simulink model "Ford_T3T6_ArchCnctnDigrm"  (R2016b)
settings: Solver=FixedStepDiscrete  StartTime=0.0  StopTime=10.0  RelTol=1e-3  EnableMultiTasking=on
libraries: canmsglib x15
(part 1 of 15)
Description:
  | T1xx system diagram for build 3
settings Model: SimulationMode=accelerator  Creator=xzs3wb  LastModifiedBy=nz3503
settings SolverCC: AutoInsertRateTranBlk=on
settings DataIOCC: LimitDataPoints=on  SaveFormat=Array  SignalLoggingSaveFormat=ModelDataLogs  SaveOutput=off  SaveTime=off
settings OptimizationCC: DefaultParameterBehavior=Inlined  InlineInvariantSignals=on  StateBitsets=on  DataBitsets=on  ZeroExternalMemoryAtStartup=off  ZeroInternalMemoryAtStartup=off  NoFixptDivByZeroProtection=on  LifeSpan=1
settings DebuggingCC: SaveWithParameterizedLinksMsg=none  UnderspecifiedInitializationDetection=Classic  MergeDetectMultiDrivingBlocksExec=none  SignalResolutionControl=TryResolveAllWithWarning  MultiTaskDSMMsg=warning  MultiTaskCondExecSysMsg=none  ParameterTunabilityLossMsg=error  StrictBusMsg=None  SFUnexpectedBacktrackingDiag=warning  SFNoUnconditionalDefaultTransitionDiag=warning  SFExecutionAtInitializationDiag=none
settings HardwareCC: ProdBitPerPointer=32  ProdBitPerSizeT=32  ProdBitPerPtrDiffT=32  ProdLargestAtomicFloat=None  ProdIntDivRoundTo=Floor  ProdWordSize=32  ProdHWDeviceType=Generic->Custom  TargetBitPerPointer=64  TargetBitPerSizeT=64  TargetBitPerPtrDiffT=64  TargetLongLongMode=on  TargetIntDivRoundTo=Zero  TargetEndianess=LittleEndian  TargetWordSize=64  TargetHWDeviceType=MATLAB Host  ProdEqTarget=off
settings ModelReferenceCC: PropagateSignalLabelsOutOfModel=off
settings RTWCC: SystemTargetFile=ert.tlc  TLCOptions=-p0  GenCodeOnly=on  TemplateMakefile=ert_default_tmf  Description=Embedded Coder  GenerateReport=on  RTWVerbose=off  IncludeHyperlinkInReport=on  LaunchReport=on  GenerateTraceInfo=on  GenerateTraceReport=on  GenerateTraceReportSl=on  GenerateTraceReportSf=on  GenerateTraceReportEml=on
settings CodeAppCC: ForceParamTrailComments=on  IgnoreCustomStorageClasses=off  OperatorAnnotations=on  SimulinkDataObjDesc=on  SFDataObjDesc=on  MATLABFcnDesc=on  CustomSymbolStrGlobalVar=rt$N$M  CustomSymbolStrType=$N$M  CustomSymbolStrFcn=$N$M$F  CustomSymbolStrMacro=$N$M  InsertBlockDesc=on  MATLABSourceComments=on
settings ERTTargetCC: CodeReplacementLibrary=ISO_C  GenerateSampleERTMain=on  IncludeMdlTerminateFcn=off  SuppressErrorStatus=on  SupportAbsoluteTime=off  SupportNonFinite=off  SupportComplex=off  PurelyIntegerCode=on  InlinedParameterPlacement=NonHierarchical  RootIOFormat=Structure reference  ERTCustomFileTemplate=example_file_process.tlc
settings ConfigComp: CovMetricSettings=dw  CovHtmlReporting=on  CovSaveCumulativeToWorkspaceVar=on  CovSaveSingleToWorkspaceVar=on  CovExternalEMLEnable=off

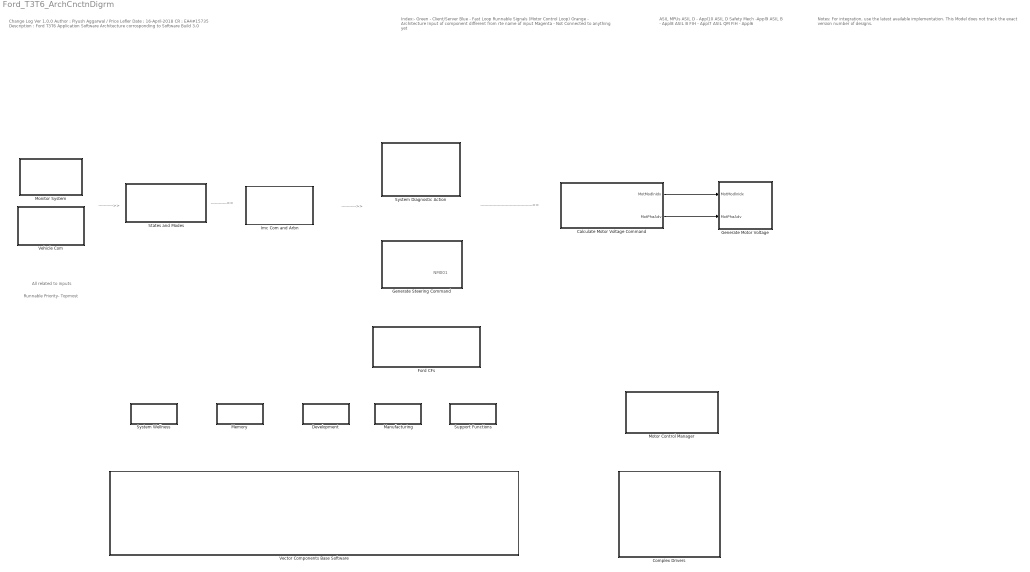
== system Ford_T3T6_ArchCnctnDigrm ==
  note: --------------------------------------->>
  note: Runnable Priority- Topmost
  note: All related to inputs
  note: ------------>>
  note: ----------->>
  note: ----------->>
  note: Change Log
      |
      | Ver 1.0.0
      | Author : Piyush Aggarwal / Price Lefler
      | Date : 16-April-2018
      | CR : EA4#15735
      | Description : Ford T3T6 Application Software Architecture corrosponding to Software Build 3.0
  note: Index:-
      |
      | Green - Client/Server
      | Blue - Fast Loop Runnable Signals (Motor Control Loop)
      | Orange - Architecture Input of component different from rte name of input
      | Magenta - Not Connected to anything yet
  note: ASIL MPUs
      |
      | ASIL D - Appl10
      | ASIL D Safety Mech -Appl9
      | ASIL B - Appl8
      | ASIL B FIH - Appl7
      | ASIL QM FIH - Appl6
  note: NM001
  note: Notes:
      | For integration, use the latest available implementation. This Model does not track the exact version number of designs.
  Calculate Motor Voltage Command : Subsystem
  Complex Drivers : Subsystem
  Development : Subsystem
  Ford CFs : Subsystem
  Generate Motor Voltage : Subsystem
  Generate Steering Command : Subsystem
  Imc Com and Arbn : Subsystem
  Manufacturing : Subsystem
  Memory : Subsystem
  Monitor System : Subsystem
  Motor Control Manager : Subsystem
  States and Modes : Subsystem
  Support Functions : Subsystem
  System Diagnostic Action : Subsystem
  System Wellness : Subsystem
  Vector Components Base Software : Subsystem
  Vehicle Com : Subsystem
  wires:
  Calculate Motor Voltage Command/1(MotModlnIdx) -> Generate Motor Voltage/1(MotModlnIdx)
  Calculate Motor Voltage Command/2(MotPhaAdv) -> Generate Motor Voltage/2(MotPhaAdv)

== system Ford_T3T6_ArchCnctnDigrm/Calculate Motor Voltage Command ==
  note: Diag Service?
  note: ASIL D
  note: ASIL D
  Motor Control : Subsystem
  SF019B_PwrLimr : Subsystem  Tag=4.0.0  Description="The purpose of the Power Limit function is to limit the system output power in a manner to enforce a desired limit on the system supply current draw.  The Power Limit function limits system output power as a function of available voltage at the inverter (DC Link Voltage) and Motor Velocity.  Additionally, a function is included to prevent excessive motor currents from being requested when the system is very hot (i.e., in Extended Operating Conditions for temperature). In additional to calculation of the Power Limit, the Power Limit Function also calculates a level of degradation from Standard Operating Conditions full performance and sets flags appropriately for a DTC (Log Only). *** PosSrvoEnable_Cnt_lgc is in documentation, but not in code. ***"
      settings: AttributesFormatString=Version: %<Tag>
  SF032A_MotTqCmdSca1 : Subsystem  Tag=1.2.3  Description=The Torque Command Scale function multiplies the MRF Motor Torque Commandinput signal by a calibration which is set during a manufacturing end of line calibration process. The calibration is provided to reduce overall system outputtorque variation. This scaled version of the motor torque command is used by SF99B - Motor control
      settings: AttributesFormatString=Version: %<Tag>
  SF050A_MotTqTranlDampg : Subsystem  Tag=1.3.0  Description=Transitional damping is computed, triggered by LoaState or DiagStatus
      settings: AttributesFormatString=Version: %<Tag>
  MotModlnIdx : Outport
  MotPhaAdv : Outport  Port=2
  tag scope: GetMotTqCmdSca=global, MotTqCmdCrfDampd=global, MotTqCmdMrfScad=global, MotTqCmdPwrLimd=global, MotTqTranlDampgCmpl=global, PwrLimrRednFac=global, SetMotTqCmdSca=global
  wires:
  Motor Control/1(MotModlnIdx) -> MotModlnIdx/1
  Motor Control/2(MotPhaAdv) -> MotPhaAdv/1
  [AltFltActv] -> SF019B_PwrLimr/1(AltFltActv)
  [BrdgVltg] -> SF019B_PwrLimr/2(BrdgVltg)
  [DualEcuFltMtgtnSca] -> SF019B_PwrLimr/3(DualEcuFltMtgtnSca)
  [MotAndThermProtnLoaMod] -> SF019B_PwrLimr/4(MotAndThermProtnLoaMod)
  [MotBackEmfConEstimd] -> SF019B_PwrLimr/5(MotBackEmfConEstimd)
  SF050A_MotTqTranlDampg/2(MotTqCmdMrfDampd) -> SF019B_PwrLimr/6(MotTqCmdMrf)
  [MotVelMrf] -> SF019B_PwrLimr/7(MotVelMrf)
  [GetRefTmr100MicroSec32bit] -> SF019B_PwrLimr/8(GetRefTmr100MicroSec32bit)
  [GetTiSpan100MicroSec32bit] -> SF019B_PwrLimr/9(GetTiSpan100MicroSec32bit)
  [SetNtcSts10] -> SF019B_PwrLimr/10(SetNtcSts)
  SF019B_PwrLimr/2(PwrLimrRednFac) -> [PwrLimrRednFac]
  SF019B_PwrLimr/1(MotTqCmdPwrLimd) -> [MotTqCmdPwrLimd], SF032A_MotTqCmdSca1/1(MotTqCmdMrf)
  [NvMProxy_GetErrorStatus] -> SF032A_MotTqCmdSca1/2(MotTqScaFac_GetErrorStatus)
  [NvMProxy_SetRamBlockStatus] -> SF032A_MotTqCmdSca1/3(MotTqScaFac_SetRamBlockStatus)
  SF032A_MotTqCmdSca1/1(MotTqCmdMrfScad) -> Motor Control/1(MotTqCmdMrfFinal), [MotTqCmdMrfScad]
  SF032A_MotTqCmdSca1/2(GetMotTqCmdSca) -> [GetMotTqCmdSca]
  SF032A_MotTqCmdSca1/3(SetMotTqCmdSca) -> [SetMotTqCmdSca]
  [AssiMechPolarity] -> SF050A_MotTqTranlDampg/1(AssiMechPolarity)
  [DiagcStsCtrldShtDwnFltPrsnt] -> SF050A_MotTqTranlDampg/2(DiagcStsCtrldShtDwnFltPrsnt)
  [HwAg] -> SF050A_MotTqTranlDampg/3(HwAg)
  [LoaSt] -> SF050A_MotTqTranlDampg/4(LoaSt)
  [MotTqCmdSwp] -> SF050A_MotTqTranlDampg/5(MotTqCmdCrf)
  [MotVelCrf] -> SF050A_MotTqTranlDampg/6(MotVelCrf)
  [SysSt] -> SF050A_MotTqTranlDampg/7(SysSt)
  [VehSpd] -> SF050A_MotTqTranlDampg/8(VehSpd)
  [GetRefTmr100MicroSec32bit] -> SF050A_MotTqTranlDampg/9(GetRefTmr100MicroSec32bit)
  [GetTiSpan100MicroSec32bit] -> SF050A_MotTqTranlDampg/10(GetTiSpan100MicroSec32bit)
  SF050A_MotTqTranlDampg/1(MotTqCmdCrfDampd) -> [MotTqCmdCrfDampd]
  SF050A_MotTqTranlDampg/3(MotTqTranlDampgCmpl) -> [MotTqTranlDampgCmpl]

== system Ford_T3T6_ArchCnctnDigrm/Complex Drivers ==
  note: ASIL D Safety Mech.
  note: ASIL D Safety Mech.
  note: ASIL D
  note: ASIL D Safety Mech.
  note: ASIL D
  AR102B_NxtrTi : Subsystem  Tag=1.0.0  Description=Nexteer Time Library
      settings: AttributesFormatString=Version: %<Tag>
  CM101B_ExcpnHndlg : Subsystem  Tag=1.2.0  Description=Handles exceptions, FE server functions and sets pre OS start up faults
      settings: AttributesFormatString=Version: %<Tag>
  CM102B_FlsMem : Subsystem  Tag=1.1.0  Description=Code Flash memory diagnostics
      settings: AttributesFormatString=Version: %<Tag>
  CM103B_RamMem : Subsystem  Tag=1.1.0  Description=Diagnostics related to RAM memory - Local, periperal and I-Cache
      settings: AttributesFormatString=Version: %<Tag>
  CM104B_EcmOutpAndDiagc : Subsystem  Tag=1.2.0  Description=Manual control over error out pin (ERROROUTZ) and startup verification test of ECM Master/Checker functionality
      settings: AttributesFormatString=Version: %<Tag>
  CM106B_McuCoreCfgAndDiagc : Subsystem  Tag=1.1.0  Description=This function describes some of the basic MCU diagnostics of the RH850/P1MC microcontroller Field BIST (built-in self-test)
      settings: AttributesFormatString=Version: %<Tag>
  CM109B_ClkCfgAndMon : Subsystem  Tag=1.1.0  Description=Nexteer Clock Monitor Config And Use
      settings: AttributesFormatString=Version: %<Tag>
  CM800A_SyncCrc : Subsystem  Tag=1.2.0  Description=CM800A provides an API for software components to run synchronous CRC calculations with the hardware CRC units on the EA4 micro controller
      settings: AttributesFormatString=Version: %<Tag>
  ES104B_XcpIf : Subsystem  Tag=0.0.0  Description=[ ]
      settings: AttributesFormatString=Version: %<Tag>
  Ford001A_ChkPt : Subsystem  Tag=0.0.0  Description=Check Point Supports alive monitoring and program flow monitoring
      settings: AttributesFormatString=Version: %<Tag>
  Platform Config : Subsystem
  tag scope: Calc16BitCrc_u08=global, Calc16BitCrc_u16=global, Calc32BitCrc_u08=global, Calc32BitCrc_u16=global, Calc32BitCrc_u32=global, Calc8BitCrc0X2F=global, Calc8BitCrc=global, ChkForStrtUpTest=global, CodFlsCrcChkCmpl=global, CtrlErrOut=global, FeNmiBusBrdgErr=global, FeNmiBusSngBitEccErr=global, FeNmiClkMonr0RtErr=global, FeNmiClkMonr1RtErr=global, FeNmiClkMonr2RtErr=global, FeNmiClkMonr3RtErr=global, FeNmiClkMonr5RtErr=global, FeNmiCodFlsEccAdrOvfErr=global, FeNmiCodFlsIllglAcsBySysBus=global, FeNmiDmaIllglAcsErr=global, FeNmiDmaLockStepErrOrGblRamWrBufErr=global, FeNmiDmaTrfErr=global, FeNmiDtsRamDblBitEccErr=global, FeNmiEcmMstChkrErr=global, FeNmiFlsSeqErr=global, FeNmiGblRamIllglAcsByProcr=global, FeNmiGblRamIllglAcsBySysBus=global, FeNmiGlbRamEccAdrOvfErr=global, FeNmiGtmRamDblBitEccErr=global, FeNmiLclRamEccAdrOvfErr=global, FeNmiModErrDbgActv=global, FeNmiModErrProgmModActv=global, FeNmiModErrTestModActv=global, FeNmiModErrUsrModInactv=global, FeNmiPegErr=global, FeNmiProcrLockStepErr=global, FeNmiPrphlRamEccAdrOvfErr=global, FeNmiResdAreaIllglAcsByHiSpdBus=global, FeNmiWdgErr=global, GetMcuDiagcIdnData=global, GetMcuDiagcSpplData=global, GetRefTmr100MicroSec32bit=global, GetRefTmr1MicroSec32bit=global, GetTiSpan100MicroSec32bit=global, GetTiSpan1MicroSec32bit=global, GlbRamEccSngBitCntrOutp=global, LclRamEccSngBitCntrOutp=global, ProcMpuExcpnErr=global, ProcNonCritOsErr=global, ProcPrmntOsErr=global, ProcPrvlgdInstrExcpnErr=global, ProcUkwnExcpnErr=global, ResvCrcHwUnit=global, SetMcuDiagcIdnData=global, SwApplCrc=global
  wires:
  [ChkForStrtUpTest] -> CM102B_FlsMem/1(ChkForStrtUpTest)
  [GetRefTmr100MicroSec32bit] -> CM102B_FlsMem/2(GetRefTmr100MicroSec32bit)
  [GetTiSpan100MicroSec32bit] -> CM102B_FlsMem/3(GetTiSpan100MicroSec32bit)
  [ResvCrcHwUnit] -> CM102B_FlsMem/4(ResvCrcHwUnit)
  [SetNtcSts] -> CM102B_FlsMem/5(SetNtcSts)
  CM102B_FlsMem/1(CodFlsCrcChkCmpl) -> [CodFlsCrcChkCmpl]
  CM102B_FlsMem/2(SwApplCrc) -> [SwApplCrc]
  CM800A_SyncCrc/1(Calc16BitCrc_u08) -> [Calc16BitCrc_u08]
  CM800A_SyncCrc/2(Calc16BitCrc_u16) -> [Calc16BitCrc_u16]
  CM800A_SyncCrc/3(Calc32BitCrc_u08) -> [Calc32BitCrc_u08]
  CM800A_SyncCrc/4(Calc32BitCrc_u16) -> [Calc32BitCrc_u16]
  CM800A_SyncCrc/5(Calc32BitCrc_u32) -> [Calc32BitCrc_u32]
  CM800A_SyncCrc/6(Calc8BitCrc) -> [Calc8BitCrc]
  CM800A_SyncCrc/7(Calc8BitCrc0X2F) -> [Calc8BitCrc0X2F]
  CM800A_SyncCrc/8(ResvCrcHwUnit) -> [ResvCrcHwUnit]
  [GetMcuDiagcIdnData] -> CM106B_McuCoreCfgAndDiagc/1(GetMcuDiagcIdnData)
  [SetMcuDiagcIdnData] -> CM106B_McuCoreCfgAndDiagc/2(SetMcuDiagcIdnData)
  [ChkForStrtUpTest] -> CM104B_EcmOutpAndDiagc/1(ChkForStrtUpTest)
  [GetMcuDiagcIdnData] -> CM104B_EcmOutpAndDiagc/2(GetMcuDiagcIdnData)
  [SetMcuDiagcIdnData] -> CM104B_EcmOutpAndDiagc/3(SetMcuDiagcIdnData)
  CM104B_EcmOutpAndDiagc/1(CtrlErrOut) -> [CtrlErrOut]
  [SetNtcSts] -> CM103B_RamMem/1(SetNtcSts)
  CM103B_RamMem/1(GlbRamEccSngBitCntrOutp) -> [GlbRamEccSngBitCntrOutp]
  CM103B_RamMem/2(LclRamEccSngBitCntrOutp) -> [LclRamEccSngBitCntrOutp]
  [SetNtcSts] -> CM101B_ExcpnHndlg/1(SetNtcSts)
  [SetNtcStsAndSnpshtData9] -> CM101B_ExcpnHndlg/2(SetNtcStsAndSnpshtData)
  CM101B_ExcpnHndlg/1(ChkForStrtUpTest) -> [ChkForStrtUpTest]
  CM101B_ExcpnHndlg/2(FeNmiBusBrdgErr) -> [FeNmiBusBrdgErr]
  CM101B_ExcpnHndlg/3(FeNmiBusSngBitEccErr) -> [FeNmiBusSngBitEccErr]
  CM101B_ExcpnHndlg/4(FeNmiClkMonr0RtErr) -> [FeNmiClkMonr0RtErr]
  CM101B_ExcpnHndlg/5(FeNmiClkMonr1RtErr) -> [FeNmiClkMonr1RtErr]
  CM101B_ExcpnHndlg/6(FeNmiClkMonr2RtErr) -> [FeNmiClkMonr2RtErr]
  CM101B_ExcpnHndlg/7(FeNmiClkMonr3RtErr) -> [FeNmiClkMonr3RtErr]
  CM101B_ExcpnHndlg/8(FeNmiClkMonr5RtErr) -> [FeNmiClkMonr5RtErr]
  CM101B_ExcpnHndlg/9(FeNmiCodFlsEccAdrOvfErr) -> [FeNmiCodFlsEccAdrOvfErr]
  CM101B_ExcpnHndlg/10(FeNmiCodFlsIllglAcsBySysBus) -> [FeNmiCodFlsIllglAcsBySysBus]
  CM101B_ExcpnHndlg/11(FeNmiDmaIllglAcsErr) -> [FeNmiDmaIllglAcsErr]
  CM101B_ExcpnHndlg/12(FeNmiDmaLockStepErrOrGblRamWrBufErr) -> [FeNmiDmaLockStepErrOrGblRamWrBufErr]
  CM101B_ExcpnHndlg/13(FeNmiDmaTrfErr) -> [FeNmiDmaTrfErr]
  CM101B_ExcpnHndlg/14(FeNmiDtsRamDblBitEccErr) -> [FeNmiDtsRamDblBitEccErr]
  CM101B_ExcpnHndlg/15(FeNmiEcmMstChkrErr) -> [FeNmiEcmMstChkrErr]
  CM101B_ExcpnHndlg/16(FeNmiFlsSeqErr) -> [FeNmiFlsSeqErr]
  CM101B_ExcpnHndlg/17(FeNmiGblRamIllglAcsByProcr) -> [FeNmiGblRamIllglAcsByProcr]
  CM101B_ExcpnHndlg/18(FeNmiGblRamIllglAcsBySysBus) -> [FeNmiGblRamIllglAcsBySysBus]
  CM101B_ExcpnHndlg/19(FeNmiGlbRamEccAdrOvfErr) -> [FeNmiGlbRamEccAdrOvfErr]
  CM101B_ExcpnHndlg/20(FeNmiGtmRamDblBitEccErr) -> [FeNmiGtmRamDblBitEccErr]
  CM101B_ExcpnHndlg/21(FeNmiLclRamEccAdrOvfErr) -> [FeNmiLclRamEccAdrOvfErr]
  CM101B_ExcpnHndlg/22(FeNmiModErrDbgActv) -> [FeNmiModErrDbgActv]
  CM101B_ExcpnHndlg/23(FeNmiModErrProgmModActv) -> [FeNmiModErrProgmModActv]
  CM101B_ExcpnHndlg/24(FeNmiModErrTestModActv) -> [FeNmiModErrTestModActv]
  CM101B_ExcpnHndlg/25(FeNmiModErrUsrModInactv) -> [FeNmiModErrUsrModInactv]
  CM101B_ExcpnHndlg/26(FeNmiPegErr) -> [FeNmiPegErr]
  CM101B_ExcpnHndlg/27(FeNmiProcrLockStepErr) -> [FeNmiProcrLockStepErr]
  CM101B_ExcpnHndlg/28(FeNmiPrphlRamEccAdrOvfErr) -> [FeNmiPrphlRamEccAdrOvfErr]
  CM101B_ExcpnHndlg/29(FeNmiResdAreaIllglAcsByHiSpdBus) -> [FeNmiResdAreaIllglAcsByHiSpdBus]
  CM101B_ExcpnHndlg/30(FeNmiWdgErr) -> [FeNmiWdgErr]
  CM101B_ExcpnHndlg/31(GetMcuDiagcIdnData) -> [GetMcuDiagcIdnData]
  CM101B_ExcpnHndlg/32(GetMcuDiagcSpplData) -> [GetMcuDiagcSpplData]
  CM101B_ExcpnHndlg/33(ProcMpuExcpnErr) -> [ProcMpuExcpnErr]
  CM101B_ExcpnHndlg/34(ProcNonCritOsErr) -> [ProcNonCritOsErr]
  CM101B_ExcpnHndlg/35(ProcPrmntOsErr) -> [ProcPrmntOsErr]
  CM101B_ExcpnHndlg/36(ProcPrvlgdInstrExcpnErr) -> [ProcPrvlgdInstrExcpnErr]
  CM101B_ExcpnHndlg/37(ProcUkwnExcpnErr) -> [ProcUkwnExcpnErr]
  CM101B_ExcpnHndlg/38(SetMcuDiagcIdnData) -> [SetMcuDiagcIdnData]
  [ClrErrInjReg] -> AR102B_NxtrTi/1(ClrErrInjReg)
  [ReadErrInjReg] -> AR102B_NxtrTi/2(ReadErrInjReg)
  [SetNtcSts10] -> AR102B_NxtrTi/3(SetNtcSts)
  AR102B_NxtrTi/1(GetRefTmr100MicroSec32bit) -> [GetRefTmr100MicroSec32bit]
  AR102B_NxtrTi/2(GetRefTmr1MicroSec32bit) -> [GetRefTmr1MicroSec32bit]
  AR102B_NxtrTi/3(GetTiSpan100MicroSec32bit) -> [GetTiSpan100MicroSec32bit]
  AR102B_NxtrTi/4(GetTiSpan1MicroSec32bit) -> [GetTiSpan1MicroSec32bit]

== system Ford_T3T6_ArchCnctnDigrm/Development ==
  note: ASIL B
  DF001A_FltInj : Subsystem  Tag=2.3.0  Description="This function injects custom values into a desired signal path.  The values to be injected are obtained via CANape interface and can take the form of a sinusoid, boolean value, integer value, or gain & offset applied to a floating point signal."
      settings: AttributesFormatString=Version: %<Tag>
  tag scope: FltInj_f32=global, FltInj_logl=global, FltInj_u08=global, FltInj_u0p16=global
  wires:
  [HwVel] -> DF001A_FltInj/1(HwVel)
  [GetRefTmr100MicroSec32bit] -> DF001A_FltInj/2(GetRefTmr100MicroSec32bit)
  [GetTiSpan100MicroSec32bit] -> DF001A_FltInj/3(GetTiSpan100MicroSec32bit)
  DF001A_FltInj/1(FltInj_f32) -> [FltInj_f32]
  DF001A_FltInj/2(FltInj_logl) -> [FltInj_logl]
  DF001A_FltInj/3(FltInj_u08) -> [FltInj_u08]
  DF001A_FltInj/4(FltInj_u0p16) -> [FltInj_u0p16]

== system Ford_T3T6_ArchCnctnDigrm/Ford CFs ==
  note: May be needed to calculate the data which will be fed to CF086
  note: Not Yet Added:-
  note: CF087A
  note: // Write --> data flow from FIH to nexteer
  note: // Read --> The Vehicle Physical Parameters (e.g. Wheelbase, Rack-to-Pinion Ratio, etc.) must be provided by Base EPS to In-House Features via Software
      | Read Functions. In-House Features that require these parameters will request it once during Initialization.
  Customer Diag Services : Subsystem
  FIH Read and Write : Subsystem
  Internal CF : Subsystem

== system Ford_T3T6_ArchCnctnDigrm/Generate Motor Voltage ==
  note: From AR300
  note: ASIL D
  note: ASIL D
  MotModlnIdx : Inport
  MotPhaAdv : Inport  Port=2
  CM770A_GtmCfgAndUse : Subsystem  Tag=2.5.0  Description=Peripheral Gtm Configuration and Use
      settings: AttributesFormatString=Version: %<Tag>
  ES300A_SinVltgGenn : Subsystem  Tag=2.4.0  Description=Sine Voltage Generation
      settings: AttributesFormatString=Version: %<Tag>
  Terminator1 : Terminator
  tag scope: GtmGetSent0Data=global, GtmGetSent1Data=global, MotCtrlCmuOffs=global, MotCtrlPhaOnTiA=global, MotCtrlPhaOnTiB=global, MotCtrlPhaOnTiC=global, MotCtrlPhaOnTiSumA=global, MotCtrlPhaOnTiSumB=global, MotCtrlPhaOnTiSumC=global, MotCtrlPwmPerd=global, PhaOnTiMeasdA=global, PhaOnTiMeasdB=global, PhaOnTiMeasdC=global
  wires:
  [MotCurrEolCalSt] -> CM770A_GtmCfgAndUse/1(MotCurrEolCalSt)
  [SysSt] -> CM770A_GtmCfgAndUse/2(SysSt)
  [MotCtrlMotCurrEolCalSt] -> CM770A_GtmCfgAndUse/3(MotCtrlMotCurrEolCalSt)
  ES300A_SinVltgGenn/2(MotCtrlPhaOnTiA) -> CM770A_GtmCfgAndUse/4(MotCtrlPhaOnTiA), [MotCtrlPhaOnTiA]
  ES300A_SinVltgGenn/3(MotCtrlPhaOnTiB) -> CM770A_GtmCfgAndUse/5(MotCtrlPhaOnTiB), [MotCtrlPhaOnTiB]
  ES300A_SinVltgGenn/4(MotCtrlPhaOnTiC) -> CM770A_GtmCfgAndUse/6(MotCtrlPhaOnTiC), [MotCtrlPhaOnTiC]
  ES300A_SinVltgGenn/8(MotCtrlPwmPerd) -> CM770A_GtmCfgAndUse/7(MotCtrlPwmPerd), [MotCtrlPwmPerd]
  [IoHwAb_SetFctGpioPhaALowrCmd] -> CM770A_GtmCfgAndUse/8(IoHwAb_SetFctGpioPhaALowrCmd)
  [IoHwAb_SetFctGpioPhaAUpprCmd] -> CM770A_GtmCfgAndUse/9(IoHwAb_SetFctGpioPhaAUpprCmd)
  [IoHwAb_SetFctGpioPhaBLowrCmd] -> CM770A_GtmCfgAndUse/10(IoHwAb_SetFctGpioPhaBLowrCmd)
  [IoHwAb_SetFctGpioPhaBUpprCmd] -> CM770A_GtmCfgAndUse/11(IoHwAb_SetFctGpioPhaBUpprCmd)
  [IoHwAb_SetFctGpioPhaCLowrCmd] -> CM770A_GtmCfgAndUse/12(IoHwAb_SetFctGpioPhaCLowrCmd)
  [IoHwAb_SetFctGpioPhaCUpprCmd] -> CM770A_GtmCfgAndUse/13(IoHwAb_SetFctGpioPhaCUpprCmd)
  [IoHwAb_SetFctPrphlPhaALowrCmd] -> CM770A_GtmCfgAndUse/14(IoHwAb_SetFctPeriphPhaALowrCmd)
  [IoHwAb_SetFctPrphlPhaAUpprCmd] -> CM770A_GtmCfgAndUse/15(IoHwAb_SetFctPeriphPhaAUpprCmd)
  [IoHwAb_SetFctPrphlPhaBLowrCmd] -> CM770A_GtmCfgAndUse/16(IoHwAb_SetFctPeriphPhaBLowrCmd)
  [IoHwAb_SetFctPrphlPhaBUpprCmd] -> CM770A_GtmCfgAndUse/17(IoHwAb_SetFctPeriphPhaBUpprCmd)
  [IoHwAb_SetFctPrphlPhaCLowrCmd] -> CM770A_GtmCfgAndUse/18(IoHwAb_SetFctPeriphPhaCLowrCmd)
  [IoHwAb_SetFctPrphlPhaCUpprCmd] -> CM770A_GtmCfgAndUse/19(IoHwAb_SetFctPeriphPhaCUpprCmd)
  [IoHwAb_SetGpioPhaALowrCmd] -> CM770A_GtmCfgAndUse/20(IoHwAb_SetGpioPhaALowrCmd)
  [IoHwAb_SetGpioPhaAUpprCmd] -> CM770A_GtmCfgAndUse/21(IoHwAb_SetGpioPhaAUpprCmd)
  [IoHwAb_SetGpioPhaBLowrCmd] -> CM770A_GtmCfgAndUse/22(IoHwAb_SetGpioPhaBLowrCmd)
  [IoHwAb_SetGpioPhaBUpprCmd] -> CM770A_GtmCfgAndUse/23(IoHwAb_SetGpioPhaBUpprCmd)
  [IoHwAb_SetGpioPhaCLowrCmd] -> CM770A_GtmCfgAndUse/24(IoHwAb_SetGpioPhaCLowrCmd)
  [IoHwAb_SetGpioPhaCUpprCmd] -> CM770A_GtmCfgAndUse/25(IoHwAb_SetGpioPhaCUpprCmd)
  CM770A_GtmCfgAndUse/1(PhaOnTiMeasdA) -> [PhaOnTiMeasdA]
  CM770A_GtmCfgAndUse/2(PhaOnTiMeasdB) -> [PhaOnTiMeasdB]
  CM770A_GtmCfgAndUse/3(PhaOnTiMeasdC) -> [PhaOnTiMeasdC]
  CM770A_GtmCfgAndUse/4(GtmGetSent0Data) -> [GtmGetSent0Data]
  CM770A_GtmCfgAndUse/5(GtmGetSent1Data) -> [GtmGetSent1Data]
  [MotElecMeclPolarity] -> ES300A_SinVltgGenn/1(MotElecMeclPolarity)
  [MotCtrlIvtrFetFltPha] -> ES300A_SinVltgGenn/2(MotCtrlIvtrFetFltPha)
  [MotCtrlIvtrFetFltTyp] -> ES300A_SinVltgGenn/3(MotCtrlIvtrFetFltTyp)
  [MotCtrlMfgEnaSt] -> ES300A_SinVltgGenn/4(MotCtrlMfgEnaSt)
  [MotCtrlMotAgElec] -> ES300A_SinVltgGenn/5(MotCtrlMotAgElec)
  MotModlnIdx/1 -> ES300A_SinVltgGenn/6(MotCtrlMotModlnIdx)
  MotPhaAdv/1 -> ES300A_SinVltgGenn/7(MotCtrlMotPhaAdv)
  [MotCtrlSwCalEna] -> ES300A_SinVltgGenn/8(MotCtrlSwCalEna)
  [MotCtrlSwCalModlnIdx] -> ES300A_SinVltgGenn/9(MotCtrlSwCalModlnIdx)
  [MotCtrlSwCalPosnIdx] -> ES300A_SinVltgGenn/10(MotCtrlSwCalPosnIdx)
  [MotCtrlVehSpd] -> ES300A_SinVltgGenn/11(MotCtrlVehSpd)
  ES300A_SinVltgGenn/1(MotCtrlCmuOffs) -> [MotCtrlCmuOffs]
  ES300A_SinVltgGenn/5(MotCtrlPhaOnTiSumA) -> [MotCtrlPhaOnTiSumA]
  ES300A_SinVltgGenn/6(MotCtrlPhaOnTiSumB) -> [MotCtrlPhaOnTiSumB]
  ES300A_SinVltgGenn/7(MotCtrlPhaOnTiSumC) -> [MotCtrlPhaOnTiSumC]

== system Ford_T3T6_ArchCnctnDigrm/Generate Steering Command ==
  note: Not actually a delay, because Swp has two 2ms runnables.
  note: ASIL B
  DF002A_Swp : Subsystem  Tag=1.8.1  Description="This function lets motor generate a sinusoidal chirp command using either a MTR (motor) configuration or HW (handwheel) configuration. This commanded input along with torque-sensor output is used for system identification of the steering gear.The Sweep function has various states. From the time sweep starts till it ends, \"sweep state\" passes throughout these states."
      settings: AttributesFormatString=Version: %<Tag>
  Openloop Steering Command : Subsystem
  tag scope: MotTqCmdSwp=global
  wires:
  Openloop Steering Command/1(MotTqCmd) -> DF002A_Swp/2(MotTqCmd)
  [HwTq] -> DF002A_Swp/1(HwTq)
  [VehSpd] -> DF002A_Swp/3(VehSpd)
  [VehSpdVld] -> DF002A_Swp/4(VehSpdVld)
  [GetRefTmr100MicroSec32bit] -> DF002A_Swp/5(GetRefTmr100MicroSec32bit)
  [GetTiSpan100MicroSec32bit] -> DF002A_Swp/6(GetTiSpan100MicroSec32bit)
  DF002A_Swp/2(MotTqCmdSwp) -> [MotTqCmdSwp]
  DF002A_Swp/1(HwTqSwp) -> Openloop Steering Command/1(HwTqSwp)

== system Ford_T3T6_ArchCnctnDigrm/Imc Com and Arbn ==
  note: ASIL D Safety Mech
  note: ASIL B
  note: ASIL B
  note: ASIL D
  note: ASIL B
  note: ASIL D
  AR350A_ImcArbn : Subsystem  Tag=1.5.0  Description=IMC Arbitration responsible to transmit, receive data between two micro controllers in a dual micro platform
      settings: AttributesFormatString=Version: %<Tag>
  CM760A_Uart0CfgAndUse : Subsystem  Tag=1.2.0  Description=Uart0 Configuration And Use Function
      settings: AttributesFormatString=Version: %<Tag>
  CM765A_Uart1CfgAndUse : Subsystem  Tag=1.2.0  Description=Uart1 Configuration And Use Function
      settings: AttributesFormatString=Version: %<Tag>
  ES011A_DualEcuIdn : Subsystem  Tag=1.3.1  Description=Identify ECU and Diagnostic
      settings: AttributesFormatString=Version: %<Tag>
  Ground : Ground
  Ground18 : Ground
  SF062B_DualCtrlrOutpMgr : Subsystem  Tag=1.0.0  Description=This function provides the ability to scale the outputof the individual ECUs in a dual ECU structure. This functionshall ensure fail operational functionality in an event of acontroller failure.It shall also provide functionality to power limit,motor control and temperature estimation in the event of a failure.The function handles voltage recoverable fault and prevents scaling inthat scenario. The function handles only voltage fault and Trim offset recovrable fault response is changed to igntion latch.
      settings: AttributesFormatString=Version: %<Tag>
  SF063A_ImcSigArbn : Subsystem  Tag=1.5.0  Description=This function shall define the requirements for sharing signals.It shall serve as a single function of contact to obtain informationfrom the other controller in a dual ECU structure. It shall definerequirements for arbitration of signals and integrator states to ensureperformance is ensured.
      settings: AttributesFormatString=Version: %<Tag>
  Terminator{1..7} (7 alike) : Terminator
  tag scope: DualEcuFltMtgtnEna=global, DualEcuFltMtgtnSca=global, DualEcuMotCtrlMtgtnEna=global, EcuId=global, GetSigImcDataExtdSts_f32=global, GetSigImcDataExtdSts_logl=global, GetSigImcDataExtdSts_s08=global, GetSigImcDataExtdSts_s16=global, GetSigImcDataExtdSts_s32=global, GetSigImcDataExtdSts_u08=global, GetSigImcDataExtdSts_u16=global, GetSigImcDataExtdSts_u32=global, GetSigImcData_f32=global, GetSigImcData_logl=global, GetSigImcData_s08=global, GetSigImcData_s16=global, GetSigImcData_s32=global, GetSigImcData_u08=global, GetSigImcData_u16=global, GetSigImcData_u32=global, GetTxRateGroup=global, GetTxSigGroup=global, HwAg=global, HwTq=global, ImcSysSt=global, ImcSysStVld=global, MotVelCrf=global, SetRxSigGroup=global, VehSpd=global
  wires:
  Ground18/1 -> ES011A_DualEcuIdn/1(EcuComTiOut)
  [GetSigImcData_u08] -> ES011A_DualEcuIdn/2(GetSigImcData_u08)
  [IoHwAb_GetGpioEcuIdnPin1] -> ES011A_DualEcuIdn/3(IoHwAb_GetGpioEcuIdnPin1)
  [IoHwAb_GetGpioEcuIdnPin2] -> ES011A_DualEcuIdn/4(IoHwAb_GetGpioEcuIdnPin2)
  [SetNtcSts10] -> ES011A_DualEcuIdn/5(SetNtcSts)
  ES011A_DualEcuIdn/1(EcuId) -> [EcuId]
  [GetTxRateGroup] -> CM760A_Uart0CfgAndUse/1(GetTxRateGroup)
  [SetRxSigGroup] -> CM760A_Uart0CfgAndUse/2(SetRxSigGroup)
  [GetTxRateGroup] -> CM765A_Uart1CfgAndUse/1(GetTxRateGroup)
  [SetRxSigGroup] -> CM765A_Uart1CfgAndUse/2(SetRxSigGroup)
  [EcuId] -> SF063A_ImcSigArbn/1(EcuIdn)
  [FordCmpdHwPosn] -> SF063A_ImcSigArbn/2(HwAg)
  [HwTqArbn] -> SF063A_ImcSigArbn/3(HwTq)
  [MotVelCrfImcInp] -> SF063A_ImcSigArbn/4(MotVelCrf)
  [PosnServoHwAg] -> SF063A_ImcSigArbn/5(PosnServoHwAg)
  [PosnServoIntgtrSt] -> SF063A_ImcSigArbn/6(PosnServoIntgtrSt)
  Ground/1 -> SF063A_ImcSigArbn/8(PosnTrakgIntgtrSt2), SF063A_ImcSigArbn/7(PosnTrakgIntgtrSt1), SF063A_ImcSigArbn/10(PullCmpShoTermIntgtrSt), SF063A_ImcSigArbn/9(PullCmpLongTermIntgtrSt)
  [VehSpdSigCdnd] -> SF063A_ImcSigArbn/11(VehSpd)
  [GetRefTmr100MicroSec32bit] -> SF063A_ImcSigArbn/12(GetRefTmr100MicroSec32bit)
  [GetSigImcData_f32] -> SF063A_ImcSigArbn/13(GetSigImcData_f32)
  [GetSigImcData_logl] -> SF063A_ImcSigArbn/14(GetSigImcData_logl)
  [GetSigImcData_u08] -> SF063A_ImcSigArbn/15(GetSigImcData_u08)
  [GetTiSpan100MicroSec32bit] -> SF063A_ImcSigArbn/16(GetTiSpan100MicroSec32bit)
  [SetNtcSts9] -> SF063A_ImcSigArbn/17(SetNtcSts)
  SF063A_ImcSigArbn/1(HwAgImcCorrd) -> [HwAg]
  SF063A_ImcSigArbn/2(HwTqImcCorrd) -> [HwTq]
  SF063A_ImcSigArbn/3(ImcSysSt) -> [ImcSysSt]
  SF063A_ImcSigArbn/4(ImcSysStVld) -> [ImcSysStVld]
  SF063A_ImcSigArbn/5(MotVelCrfImcCorrd) -> [MotVelCrf]
  SF063A_ImcSigArbn/6(PosnServoHwAgImcCorrd) -> Terminator1/1
  SF063A_ImcSigArbn/7(PosnServoIntgtrOffs) -> Terminator2/1
  SF063A_ImcSigArbn/8(PosnTrakgArbnFltMtgtnEna) -> Terminator3/1
  SF063A_ImcSigArbn/9(PosnTrakgIntgtrSt1Offs) -> Terminator4/1
  SF063A_ImcSigArbn/10(PosnTrakgIntgtrSt2Offs) -> Terminator5/1
  SF063A_ImcSigArbn/11(PullCmpLongTermIntgtrStOffs) -> Terminator6/1
  SF063A_ImcSigArbn/12(PullCmpShoTermIntgtrStOffs) -> Terminator7/1
  SF063A_ImcSigArbn/13(VehSpdImcCorrd) -> [VehSpd]
  [ImcSysSt] -> SF062B_DualCtrlrOutpMgr/1(ImcSysSt)
  [ImcSysStVld] -> SF062B_DualCtrlrOutpMgr/2(ImcSysStVld)
  [MotAndThermProtnLoaMod] -> SF062B_DualCtrlrOutpMgr/3(MotAndThermProtnLoaMod)
  [SysSt] -> SF062B_DualCtrlrOutpMgr/4(SysSt)
  [VehSpd] -> SF062B_DualCtrlrOutpMgr/5(VehSpd)
  [GetRefTmr100MicroSec32bit] -> SF062B_DualCtrlrOutpMgr/6(GetRefTmr100MicroSec32bit)
  [GetSigImcData_logl] -> SF062B_DualCtrlrOutpMgr/7(GetSigImcData_logl)
  [GetTiSpan100MicroSec32bit] -> SF062B_DualCtrlrOutpMgr/8(GetTiSpan100MicroSec32bit)
  SF062B_DualCtrlrOutpMgr/1(DualEcuFltMtgtnEna) -> [DualEcuFltMtgtnEna]
  SF062B_DualCtrlrOutpMgr/2(DualEcuFltMtgtnSca) -> [DualEcuFltMtgtnSca]
  SF062B_DualCtrlrOutpMgr/3(DualEcuMotCtrlMtgtnEna) -> [DualEcuMotCtrlMtgtnEna]
  [SetNtcSts8] -> AR350A_ImcArbn/1(SetNtcSts)
  AR350A_ImcArbn/1(GetSigImcDataExtdSts_f32) -> [GetSigImcDataExtdSts_f32]
  AR350A_ImcArbn/2(GetSigImcDataExtdSts_logl) -> [GetSigImcDataExtdSts_logl]
  AR350A_ImcArbn/3(GetSigImcDataExtdSts_s08) -> [GetSigImcDataExtdSts_s08]
  AR350A_ImcArbn/4(GetSigImcDataExtdSts_s16) -> [GetSigImcDataExtdSts_s16]
  AR350A_ImcArbn/5(GetSigImcDataExtdSts_s32) -> [GetSigImcDataExtdSts_s32]
  AR350A_ImcArbn/6(GetSigImcDataExtdSts_u08) -> [GetSigImcDataExtdSts_u08]
  AR350A_ImcArbn/7(GetSigImcDataExtdSts_u16) -> [GetSigImcDataExtdSts_u16]
  AR350A_ImcArbn/8(GetSigImcDataExtdSts_u32) -> [GetSigImcDataExtdSts_u32]
  AR350A_ImcArbn/9(GetSigImcData_f32) -> [GetSigImcData_f32]
  AR350A_ImcArbn/10(GetSigImcData_logl) -> [GetSigImcData_logl]
  AR350A_ImcArbn/11(GetSigImcData_s08) -> [GetSigImcData_s08]
  AR350A_ImcArbn/12(GetSigImcData_s16) -> [GetSigImcData_s16]
  AR350A_ImcArbn/13(GetSigImcData_s32) -> [GetSigImcData_s32]
  AR350A_ImcArbn/14(GetSigImcData_u08) -> [GetSigImcData_u08]
  AR350A_ImcArbn/15(GetSigImcData_u16) -> [GetSigImcData_u16]
  AR350A_ImcArbn/16(GetSigImcData_u32) -> [GetSigImcData_u32]
  AR350A_ImcArbn/17(GetTxRateGroup) -> [GetTxRateGroup]
  AR350A_ImcArbn/18(GetTxSigGroup) -> [GetTxSigGroup]
  AR350A_ImcArbn/19(SetRxSigGroup) -> [SetRxSigGroup]

== system Ford_T3T6_ArchCnctnDigrm/Manufacturing ==
  note: Mfg Service
  note: ASIL D
  NM002A_CmnMfgSrvIf : Subsystem  Tag=1.1.0  Description=Nexteer manufacturing services transport layer interface
      settings: AttributesFormatString=Version: %<Tag>
  NM100A_MotVelCtrl : Subsystem  Tag=1.4.0  Description=This function provides the capability to spin EPS motor at a specified velocity.This is achieved by applying motor toque based on the difference between target motor velocity and measured motor velocity.
      settings: AttributesFormatString=Version: %<Tag>
  tag scope: ApplTpRxErrIndcn=global, ApplTpRxGetBuf=global, ApplTpRxIndcn=global, ApplTpTxCfm=global, ApplTpTxErrIndcn=global, CmnMfgSrvIfImdtTx=global, GetCtrlPrm=global, SetCtrlPrm=global, StopCtrl=global, StrtCtrl=global
  wires:
  [MfgEnaSt] -> NM002A_CmnMfgSrvIf/1(MfgEnaSt)
  [CmnMfgSrvMaiFct] -> NM002A_CmnMfgSrvIf/2(CmnMfgSrvMaiFct)
  NM002A_CmnMfgSrvIf/1(ApplTpTxErrIndcn) -> [ApplTpTxErrIndcn]
  NM002A_CmnMfgSrvIf/2(ApplTpRxErrIndcn) -> [ApplTpRxErrIndcn]
  NM002A_CmnMfgSrvIf/3(ApplTpRxGetBuf) -> [ApplTpRxGetBuf]
  NM002A_CmnMfgSrvIf/4(ApplTpRxIndcn) -> [ApplTpRxIndcn]
  NM002A_CmnMfgSrvIf/5(ApplTpTxCfm) -> [ApplTpTxCfm]
  NM002A_CmnMfgSrvIf/6(CmnMfgSrvIfImdtTx) -> [CmnMfgSrvIfImdtTx]
  [MotVelCrf] -> NM100A_MotVelCtrl/1(MotVelCrf)
  [GetRefTmr100MicroSec32bit] -> NM100A_MotVelCtrl/2(GetRefTmr100MicroSec32bit)
  [GetTiSpan100MicroSec32bit] -> NM100A_MotVelCtrl/3(GetTiSpan100MicroSec32bit)
  [SetManTqCmd] -> NM100A_MotVelCtrl/4(SetManTqCmd)
  NM100A_MotVelCtrl/1(GetCtrlPrm) -> [GetCtrlPrm]
  NM100A_MotVelCtrl/2(SetCtrlPrm) -> [SetCtrlPrm]
  NM100A_MotVelCtrl/3(StopCtrl) -> [StopCtrl]
  NM100A_MotVelCtrl/4(StrtCtrl) -> [StrtCtrl]

== system Ford_T3T6_ArchCnctnDigrm/Memory ==
  note: CMS?
  note: ASIL B
  ES006A_NvMProxy : Subsystem  Tag=1.1.X  Description=The NvMProxy provides an interface for software components outside of the application of the NvM to communicate with the NvM component.
      settings: AttributesFormatString=Version: %<Tag>
  ES400A_TunSelnMngt : Subsystem  Tag=2.0.0  Description=ES400A manages run time and initialization calibration indexes for usein system operation and online calibration activities
      settings: AttributesFormatString=Version: %<Tag>
  SF023A_TunSelnAuthy : Subsystem  Tag=1.1.1  Description=This function ensures driving conditions are appropriate to switch between calibration subsets. It compares handwheel torque and vehiclespeed to calibratable thresholds and either grants or denies a requested change in either tuning set or tuning personality.
      settings: AttributesFormatString=Version: %<Tag>
  tag scope: ActvGroup=global, ActvIninIdx=global, ActvRtIdx=global, CalCopyCmpl=global, CopyCalPageReq=global, GetCalPageReq=global, GetSegInfoReq=global, NvMProxy_ClsChkWr_Oper=global, NvMProxy_GetErrorStatus=global, NvMProxy_ReadBlock=global, NvMProxy_SetRamBlockStatus=global, NvMProxy_WriteBlock=global, OnlineTunRamAdrMpg=global, PortDefinedArgument_GetErrorStatus=global, PortDefinedArgument_ReadBlock=global, PortDefinedArgument_SetRamBlockStatus=global, PortDefinedArgument_WriteBlock=global, RtCalChgReq=global, SetCalPageReq=global, XcpCalChgReq=global
  wires:
  [HwTq] -> SF023A_TunSelnAuthy/1(HwTq)
  [HwVel] -> SF023A_TunSelnAuthy/2(HwVel)
  [TunSelnRtDi] -> SF023A_TunSelnAuthy/3(TunSelnRtDi)
  [VehSpd] -> SF023A_TunSelnAuthy/4(VehSpd)
  SF023A_TunSelnAuthy/1(RtCalChgReq) -> [RtCalChgReq]
  SF023A_TunSelnAuthy/2(XcpCalChgReq) -> [XcpCalChgReq]
  [DesIninIdx] -> ES400A_TunSelnMngt/1(DesIninIdx)
  [DesRtIdx] -> ES400A_TunSelnMngt/2(DesRtIdx)
  [Calc32BitCrc_u32] -> ES400A_TunSelnMngt/3(Calc32BitCrc_u32)
  [RtCalChgReq] -> ES400A_TunSelnMngt/4(RtCalChgReq)
  [SetNtcSts] -> ES400A_TunSelnMngt/5(SetNtcSts)
  ES400A_TunSelnMngt/1(ActvGroup) -> [ActvGroup]
  ES400A_TunSelnMngt/2(ActvIninIdx) -> [ActvIninIdx]
  ES400A_TunSelnMngt/3(ActvRtIdx) -> [ActvRtIdx]
  ES400A_TunSelnMngt/4(CalCopyCmpl) -> [CalCopyCmpl]
  ES400A_TunSelnMngt/5(CopyCalPageReq) -> [CopyCalPageReq]
  ES400A_TunSelnMngt/6(GetCalPageReq) -> [GetCalPageReq]
  ES400A_TunSelnMngt/7(GetSegInfoReq) -> [GetSegInfoReq]
  ES400A_TunSelnMngt/8(OnlineTunRamAdrMpg) -> [OnlineTunRamAdrMpg]
  ES400A_TunSelnMngt/9(SetCalPageReq) -> [SetCalPageReq]
  [NvM_GetErrorStatus] -> ES006A_NvMProxy/1(NvM_GetErrorStatus)
  [NvM_ReadBlock] -> ES006A_NvMProxy/2(NvM_ReadBlock)
  [NvM_SetRamBlockStatus] -> ES006A_NvMProxy/3(NvM_SetRamBlockStatus)
  [NvM_WriteBlock] -> ES006A_NvMProxy/4(NvM_WriteBlock)
  ES006A_NvMProxy/1(NvMProxy_ClsChkWr_Oper) -> [NvMProxy_ClsChkWr_Oper]
  ES006A_NvMProxy/2(NvMProxy_GetErrorStatus) -> [NvMProxy_GetErrorStatus]
  ES006A_NvMProxy/3(NvMProxy_ReadBlock) -> [NvMProxy_ReadBlock]
  ES006A_NvMProxy/4(NvMProxy_SetRamBlockStatus) -> [NvMProxy_SetRamBlockStatus]
  ES006A_NvMProxy/5(NvMProxy_WriteBlock) -> [NvMProxy_WriteBlock]
  ES006A_NvMProxy/6(PortDefinedArgument_GetErrorStatus) -> [PortDefinedArgument_GetErrorStatus]
  ES006A_NvMProxy/7(PortDefinedArgument_ReadBlock) -> [PortDefinedArgument_ReadBlock]
  ES006A_NvMProxy/8(PortDefinedArgument_SetRamBlockStatus) -> [PortDefinedArgument_SetRamBlockStatus]
  ES006A_NvMProxy/9(PortDefinedArgument_WriteBlock) -> [PortDefinedArgument_WriteBlock]

== system Ford_T3T6_ArchCnctnDigrm/Monitor System ==
  Inferred Signals : Subsystem
  Measured Signals : Subsystem
  wires:
  Inferred Signals/1(MotVelMrf) -> Measured Signals/1(MotVelMrf)
  Measured Signals/1(HwTq) -> Inferred Signals/1(HwTq)
  Measured Signals/2(HwAgMeas) -> Inferred Signals/2(HwAgMeas)
  Measured Signals/3(HwAgIdptSig) -> Inferred Signals/3(HwAgIdptSig)
  Measured Signals/4(MotAgMech) -> Inferred Signals/4(MotAgMecl)
  Measured Signals/5(EcuTFild) -> Inferred Signals/5(EcuTFild)
